simulink model "PI_controller_antiwindup2"  (R2023b)
settings: Solver=FixedStepAuto  StartTime=0.0  StopTime=15  FixedStep=0.01  RelTol=1e-3
settings Model: Creator=suvo  LastModifiedBy=suvo
settings SolverCC: AlgebraicLoopSolver=TrustRegion
settings DebuggingCC: UnconnectedInputMsg=warning  UnconnectedOutputMsg=warning  UnconnectedLineMsg=warning
settings ModelReferenceCC: EnableRefExpFcnMdlSchedulingChecks=on

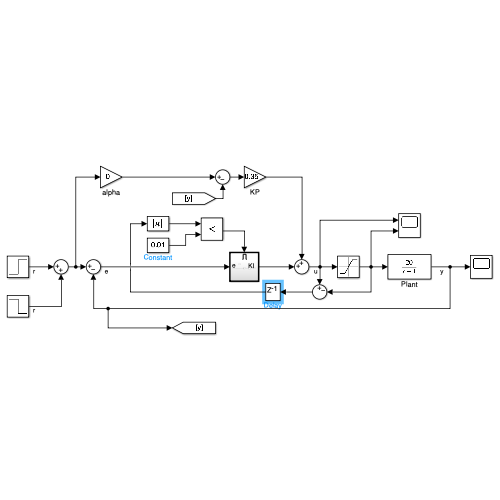
[thumbnail: Simulink's stored preview of the top-level diagram]
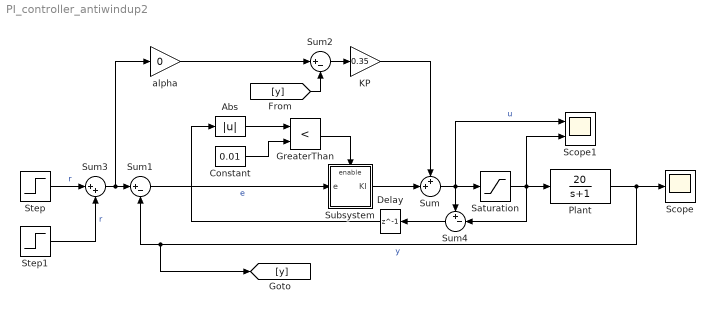
== system PI_controller_antiwindup2 ==
  Abs : Abs  SaturateOnIntegerOverflow=off
  Constant : Constant  Value=0.01
  Delay : Delay  DelayLength=1
  GreaterThan : RelationalOperator  Operator=<  OutDataTypeStr=boolean  RndMeth=Simplest  InputSameDT=off
  KP : Gain  Gain=0.35
  Plant : TransferFcn  Numerator=20  Denominator=[1 1]
  Saturation : Saturate  UpperLimit=0.03  LowerLimit=-.03
  Scope : Scope
  Scope1 : Scope  NumInputPorts=2
  Step : Step  SampleTime=0
  Step1 : Step  Time=5  After=-1  SampleTime=0
  Subsystem : Subsystem
  Sum : Sum  Inputs=++|
  Sum1 : Sum  Inputs=|+-
  Sum2 : Sum  Inputs=|+-
  Sum3 : Sum  Inputs=|++
  Sum4 : Sum  Inputs=+-|
  alpha : Gain  Gain=0
  wires:
  Plant/1 -> Scope/1, [y], Sum1/2  "y"
  Sum2/1 -> KP/1
  KP/1 -> Sum/1
  Sum/1 -> Saturation/1, Scope1/1, Sum4/1  "u"
  [y] -> Sum2/2
  alpha/1 -> Sum2/1
  Saturation/1 -> Sum4/2, Scope1/2, Plant/1
  Step/1 -> Sum3/1  "r"
  Sum3/1 -> alpha/1, Sum1/1
  Step1/1 -> Sum3/2  "r"
  Sum1/1 -> Subsystem/1(e)  "e"
  Constant/1 -> GreaterThan/2
  Subsystem/1("KI ") -> Sum/2
  Sum4/1 -> Delay/1
  Abs/1 -> GreaterThan/1
  Delay/1 -> Abs/1
  GreaterThan/1 -> Subsystem/Enable

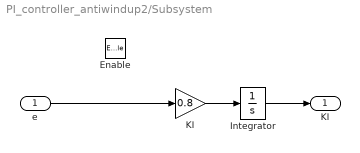
== system PI_controller_antiwindup2/Subsystem ==
  e : Inport
  Enable : EnablePort
  Integrator : Integrator  UpperSaturationLimit=0.25  LowerSaturationLimit=-0.25
  KI : Gain  Gain=0.8
  "KI " : Outport
  wires:
  e/1 -> KI/1
  KI/1 -> Integrator/1
  Integrator/1 -> "KI "/1
